simulink model "model_reg_silnik"  (R2016a)
settings: Solver=ode4  StartTime=0.0  StopTime=30  FixedStep=0.001  RelTol=1e-3
values from neighbouring files (symbols this model uses):
  A = [0  1        0       0 ... (first row only)    [obserwator.m]    (also in zad1.m = [-1 0 0 0 0)
  B = [0 (Kx + mc*R)/ Tx 0 1/R]'    [obserwator.m]    (also in zad1.m = [0 0 0 0 0]')
  C = [1 0 0 0 ... (first row only)    [obserwator.m]
  I = eye(4)    [obserwator.m]
  L = 5.93*10^(-3)    (= 0.00593)    [all2.m]    (also in cel.m; motor_x.m; motor_y.m; obserwator.m = transpose(place(transpose(A),transpose(C), [-30 -12 -11 -13])
  lin = 2    [all2.m]    (also in dane.m = 1; zad1.m = 10)
  mc = 1    [dane.m]    (also in obiekt.m; zad1.m)
  mw = X0    [celMW.m]    (also in dane.m = 1.155; obiekt.m = 1.155; zad1.m = 2.49)
  p = 60    [dane.m]    (also in zad1.m)
  reg_PD = 0    [dane.m]    (also in lsmMW.m = 1)
  x0 = [0   0   0    0   0   0    0   0   0.15   0]'    [dane.m]    (also in zad1.m)
libraries: simulink x3
settings Model: Creator=Maciek  LastModifiedBy=Maciek

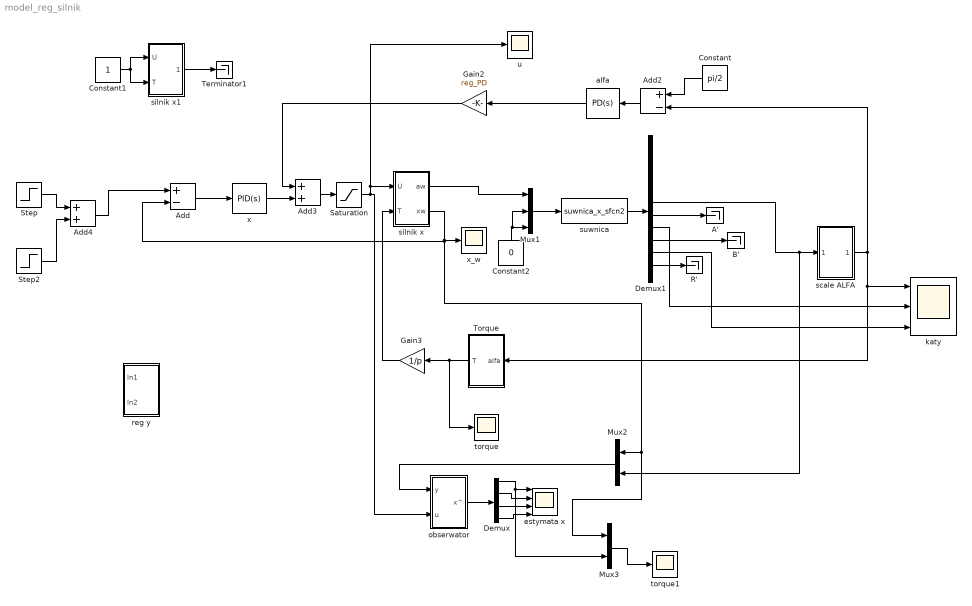
== system model_reg_silnik ==
  A' : Terminator
  Add : Sum  Inputs=+-
  Add2 : Sum  Inputs=+-
  Add3 : Sum
  Add4 : Sum
  B' : Terminator
  Constant : Constant  Value=pi/2
  Constant1 : Constant
  Constant2 : Constant  Value=0
  Demux : Demux
  Demux1 : Demux  Outputs=10
  Gain2 : Gain  Gain=reg_PD
  Gain3 : Gain  Gain=1/p
  Mux1 : Mux  Inputs=3
  Mux2 : Mux  Inputs=2
  Mux3 : Mux  Inputs=2
  R' : Terminator
  Saturation : Saturate  UpperLimit=1  LowerLimit=-1
  Step : Step  After=0.2  SampleTime=0
  Step2 : Step  Time=15  After=-0.4  SampleTime=0
  Terminator1 : Terminator
  "Torque " : Subsystem
  alfa : simulink/Continuous/PID Controller  Controller=PD  TimeDomain=Continuous-time  SampleTime=-1  IntegratorMethod=Forward Euler  FilterMethod=Forward Euler  Form=Parallel  UseFilter=on  ControllerParametersSource=internal  P=10  I=0.015  D=0.5  N=100  InitialConditionSource=internal  InitialConditionForIntegrator=0  InitialConditionForFilter=0  ExternalReset=none  LimitOutput=on  UpperSaturationLimit=1  LowerSaturationLimit=-1  LinearizeAsGain=on  AntiWindupMode=none  Kb=1  TrackingMode=off  Kt=1  PParamMin=[]  PParamMax=[]  IParamMin=[]  IParamMax=[]  DParamMin=[]  DParamMax=[]  NParamMin=[]  NParamMax=[]  KbParamMin=[]  KbParamMax=[]  KtParamMin=[]  KtParamMax=[]  POutMin=[]  POutMax=[]  IOutMin=[]  IOutMax=[]  DOutMin=[]  DOutMax=[]  NOutMin=[]  NOutMax=[]  KbOutMin=[]  KbOutMax=[]  KtOutMin=[]  KtOutMax=[]  IntegratorOutMin=[]  IntegratorOutMax=[]  FilterOutMin=[]  FilterOutMax=[]  SumOutMin=[]  SumOutMax=[]  SumI1OutMin=[]  SumI1OutMax=[]  SumI2OutMin=[]  SumI2OutMax=[]  SumI3OutMin=[]  SumI3OutMax=[]  SumDOutMin=[]  SumDOutMax=[]  SaturationOutMin=[]  SaturationOutMax=[]  IntegratorContinuousStateAttributes=''  IntegratorStateMustResolveToSignalObject=off  IntegratorRTWStateStorageClass=Auto  FilterContinuousStateAttributes=''  FilterStateMustResolveToSignalObject=off  FilterRTWStateStorageClass=Auto  DifferentiatorICPrevScaledInput=0  DifferentiatorOutMin=[]  DifferentiatorOutMax=[]
  estymata x : Scope  NumInputPorts=4
  katy : Scope  NumInputPorts=3
  obserwator : Subsystem
  reg y : Subsystem
  scale ALFA : Subsystem
  silnik x : Subsystem
  silnik x1 : Subsystem
  suwnica : S-Function  FunctionName=suwnica_x_sfcn2  Parameters=x0  SFunctionDeploymentMode=off  EnableBusSupport=off
  torque : Scope
  torque1 : Scope
  u : Scope
  x : simulink/Continuous/PID Controller  Controller=PID  TimeDomain=Continuous-time  SampleTime=-1  IntegratorMethod=Forward Euler  FilterMethod=Forward Euler  Form=Parallel  UseFilter=on  ControllerParametersSource=internal  P=10  I=0.005  D=2  N=100  InitialConditionSource=internal  InitialConditionForIntegrator=0  InitialConditionForFilter=0  ExternalReset=none  LimitOutput=on  UpperSaturationLimit=1  LowerSaturationLimit=-1  LinearizeAsGain=on  AntiWindupMode=none  Kb=1  TrackingMode=off  Kt=1  PParamMin=[]  PParamMax=[]  IParamMin=[]  IParamMax=[]  DParamMin=[]  DParamMax=[]  NParamMin=[]  NParamMax=[]  KbParamMin=[]  KbParamMax=[]  KtParamMin=[]  KtParamMax=[]  POutMin=[]  POutMax=[]  IOutMin=[]  IOutMax=[]  DOutMin=[]  DOutMax=[]  NOutMin=[]  NOutMax=[]  KbOutMin=[]  KbOutMax=[]  KtOutMin=[]  KtOutMax=[]  IntegratorOutMin=[]  IntegratorOutMax=[]  FilterOutMin=[]  FilterOutMax=[]  SumOutMin=[]  SumOutMax=[]  SumI1OutMin=[]  SumI1OutMax=[]  SumI2OutMin=[]  SumI2OutMax=[]  SumI3OutMin=[]  SumI3OutMax=[]  SumDOutMin=[]  SumDOutMax=[]  SaturationOutMin=[]  SaturationOutMax=[]  IntegratorContinuousStateAttributes=''  IntegratorStateMustResolveToSignalObject=off  IntegratorRTWStateStorageClass=Auto  FilterContinuousStateAttributes=''  FilterStateMustResolveToSignalObject=off  FilterRTWStateStorageClass=Auto  DifferentiatorICPrevScaledInput=0  DifferentiatorOutMin=[]  DifferentiatorOutMax=[]
  "x_w " : Scope
  wires:
  Mux1/1 -> suwnica/1
  Constant2/1 -> Mux1/2, Mux1/3
  Demux1/10 -> R'/1
  Demux1/8 -> B'/1
  Demux1/7 -> katy/2
  Demux1/9 -> katy/3
  Demux1/6 -> A'/1
  suwnica/1 -> Demux1/1
  Demux1/5 -> Mux2/2, scale ALFA/1(In1)
  scale ALFA/1(Out1) -> Add2/2, "Torque "/1(alfa), katy/1
  Add/1 -> x/1
  Add2/1 -> alfa/1
  Constant/1 -> Add2/1
  alfa/1 -> Gain2/1
  Add3/1 -> Saturation/1
  x/1 -> Add3/2
  Saturation/1 -> obserwator/2(u), silnik x/1(U), u/1
  Gain2/1 -> Add3/1
  "Torque "/1(T) -> torque/1, Gain3/1
  Gain3/1 -> silnik x/2(T)
  silnik x/1(aw) -> Mux1/1
  silnik x/2(xw) -> Mux3/1, Mux2/1, Add/2, "x_w "/1
  silnik x1/1(Out1) -> Terminator1/1
  Constant1/1 -> silnik x1/1(U), silnik x1/2(T)
  Mux2/1 -> obserwator/1(y)
  obserwator/1(x^) -> Demux/1
  Demux/1 -> Mux3/2, estymata x/1
  Demux/2 -> estymata x/2
  Demux/3 -> estymata x/3
  Demux/4 -> estymata x/4
  Add4/1 -> Add/1
  Step/1 -> Add4/1
  Step2/1 -> Add4/2
  Mux3/1 -> torque1/1

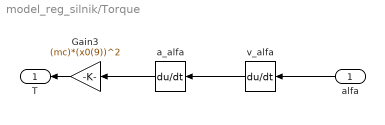
== system model_reg_silnik/Torque  ==
  alfa : Inport
  Gain3 : Gain  Gain=(mc)*(x0(9))^2
  a_alfa : Derivative
  v_alfa : Derivative
  T : Outport
  wires:
  a_alfa/1 -> Gain3/1
  alfa/1 -> v_alfa/1
  Gain3/1 -> T/1
  v_alfa/1 -> a_alfa/1

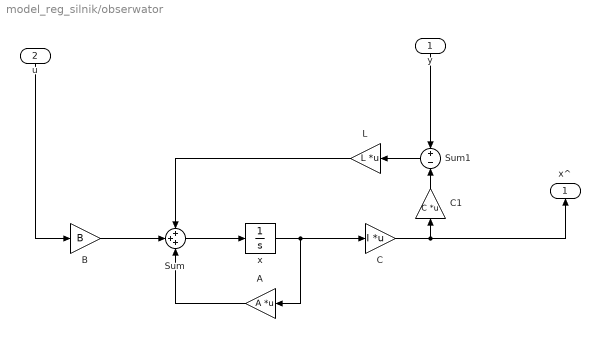
== system model_reg_silnik/obserwator ==
  y : Inport
  u : Inport  Port=2
  A : Gain  Gain=A  Multiplication=Matrix(K*u) (u vector)
  B : Gain  Gain=B
  C : Gain  Gain=I  Multiplication=Matrix(K*u) (u vector)
  C1 : Gain  Gain=C  Multiplication=Matrix(K*u) (u vector)
  L : Gain  Gain=L  Multiplication=Matrix(K*u) (u vector)
  Sum : Sum  Inputs=+++
  Sum1 : Sum  Inputs=+-
  x : Integrator  InitialCondition=[0 0 0 0]
  x^ : Outport
  wires:
  C1/1 -> Sum1/2
  y/1 -> Sum1/1
  u/1 -> B/1
  Sum/1 -> x/1
  x/1 -> A/1, C/1
  A/1 -> Sum/3
  C/1 -> x^/1, C1/1
  Sum1/1 -> L/1
  L/1 -> Sum/1
  B/1 -> Sum/2

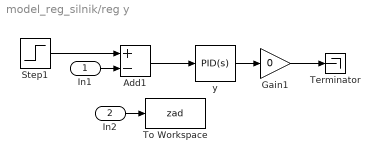
== system model_reg_silnik/reg y ==
  In1 : Inport
  In2 : Inport  Port=2
  Add1 : Sum  Inputs=+-
  Gain1 : Gain  Gain=0
  Step1 : Step  After=0  SampleTime=0
  Terminator : Terminator
  To Workspace : ToWorkspace  VariableName=zad  SaveFormat=Timeseries  SampleTime=-1
  y : simulink/Continuous/PID Controller  Controller=PID  TimeDomain=Continuous-time  SampleTime=-1  IntegratorMethod=Forward Euler  FilterMethod=Forward Euler  Form=Parallel  UseFilter=on  ControllerParametersSource=internal  P=250  I=0.002  D=1  N=100  InitialConditionSource=internal  InitialConditionForIntegrator=0  InitialConditionForFilter=0  ExternalReset=none  LimitOutput=on  UpperSaturationLimit=20  LowerSaturationLimit=-20  LinearizeAsGain=on  AntiWindupMode=none  Kb=1  TrackingMode=off  Kt=1  PParamMin=[]  PParamMax=[]  IParamMin=[]  IParamMax=[]  DParamMin=[]  DParamMax=[]  NParamMin=[]  NParamMax=[]  KbParamMin=[]  KbParamMax=[]  KtParamMin=[]  KtParamMax=[]  POutMin=[]  POutMax=[]  IOutMin=[]  IOutMax=[]  DOutMin=[]  DOutMax=[]  NOutMin=[]  NOutMax=[]  KbOutMin=[]  KbOutMax=[]  KtOutMin=[]  KtOutMax=[]  IntegratorOutMin=[]  IntegratorOutMax=[]  FilterOutMin=[]  FilterOutMax=[]  SumOutMin=[]  SumOutMax=[]  SumI1OutMin=[]  SumI1OutMax=[]  SumI2OutMin=[]  SumI2OutMax=[]  SumI3OutMin=[]  SumI3OutMax=[]  SumDOutMin=[]  SumDOutMax=[]  SaturationOutMin=[]  SaturationOutMax=[]  IntegratorContinuousStateAttributes=''  IntegratorStateMustResolveToSignalObject=off  IntegratorRTWStateStorageClass=Auto  FilterContinuousStateAttributes=''  FilterStateMustResolveToSignalObject=off  FilterRTWStateStorageClass=Auto  DifferentiatorICPrevScaledInput=0  DifferentiatorOutMin=[]  DifferentiatorOutMax=[]
  wires:
  In1/1 -> Add1/2
  In2/1 -> To Workspace/1
  y/1 -> Gain1/1
  Add1/1 -> y/1
  Step1/1 -> Add1/1
  Gain1/1 -> Terminator/1

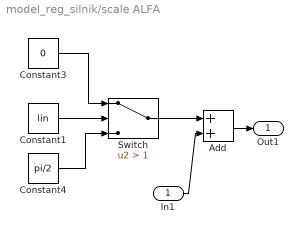
== system model_reg_silnik/scale ALFA ==
  In1 : Inport
  Add : Sum  Inputs=2
  Constant1 : Constant  Value=lin
  Constant3 : Constant  Value=0
  Constant4 : Constant  Value=pi/2
  Switch : Switch  Criteria=u2 > Threshold  Threshold=1
  Out1 : Outport
  wires:
  Add/1 -> Out1/1
  In1/1 -> Add/2
  Constant4/1 -> Switch/3
  Constant3/1 -> Switch/1
  Switch/1 -> Add/1
  Constant1/1 -> Switch/2

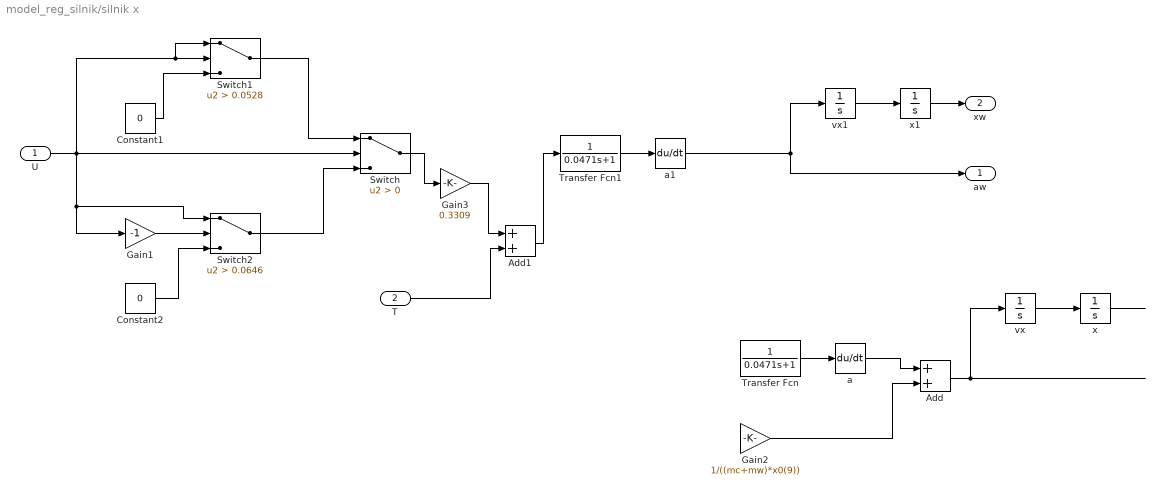
== system model_reg_silnik/silnik x ==
  U : Inport
  T : Inport  Port=2
  Add : Sum
  Add1 : Sum
  Constant1 : Constant  Value=0
  Constant2 : Constant  Value=0
  Gain1 : Gain  Gain=-1
  Gain2 : Gain  Gain=1/((mc+mw)*x0(9))
  Gain3 : Gain  Gain=0.3309
  Switch : Switch  Criteria=u2 > Threshold
  Switch1 : Switch  Criteria=u2 > Threshold  Threshold=0.0528
  Switch2 : Switch  Criteria=u2 > Threshold  Threshold=0.0646
  Transfer Fcn : TransferFcn  Numerator=1  Denominator=[0.0471 1]
  Transfer Fcn1 : TransferFcn  Numerator=1  Denominator=[0.0471 1]
  a : Derivative
  a1 : Derivative
  vx : Integrator
  vx1 : Integrator
  x : Integrator
  x1 : Integrator
  aw : Outport
  xw : Outport  Port=2
  wires:
  Constant1/1 -> Switch1/3
  Switch1/1 -> Switch/1
  Constant2/1 -> Switch2/3
  U/1 -> Switch2/1, Gain1/1, Switch1/1, Switch1/2, Switch/2
  Switch2/1 -> Switch/3
  Gain1/1 -> Switch2/2
  Transfer Fcn/1 -> a/1
  ? -> Gain2/1
  a/1 -> Add/1
  Add/1 -> vx/1
  x/1 -> ?
  vx/1 -> x/1
  Gain2/1 -> Add/2
  ? -> Transfer Fcn/1
  Transfer Fcn1/1 -> a1/1
  a1/1 -> aw/1, vx1/1
  x1/1 -> xw/1
  vx1/1 -> x1/1
  T/1 -> Add1/2
  Switch/1 -> Gain3/1
  Gain3/1 -> Add1/1
  Add1/1 -> Transfer Fcn1/1

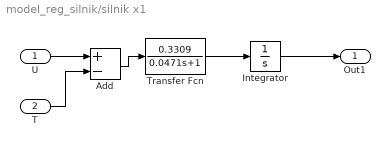
== system model_reg_silnik/silnik x1 ==
  U : Inport
  T : Inport  Port=2
  Add : Sum  Inputs=+-
  Integrator : Integrator
  Transfer Fcn : TransferFcn  Numerator=0.3309  Denominator=[0.0471 1]
  Out1 : Outport
  wires:
  Transfer Fcn/1 -> Integrator/1
  Integrator/1 -> Out1/1
  Add/1 -> Transfer Fcn/1
  U/1 -> Add/1
  T/1 -> Add/2
